simulink model "sfun_daq"  (Simulink 8.3)
settings: Solver=FixedStepDiscrete  StartTime=0.0  StopTime=inf  FixedStep=1/100  RelTol=1e-3
libraries: aerolibtransform2 x1, robotica_R2013b x1
settings Model: Creator=blazj  LastModifiedBy=blazj
settings DataIOCC: SignalLoggingSaveFormat=Dataset
settings DebuggingCC: UnderspecifiedInitializationDetection=Simplified  StateNameClashWarn=none
settings GRTTargetCC: CombineOutputUpdateFcns=on  GRTInterface=off

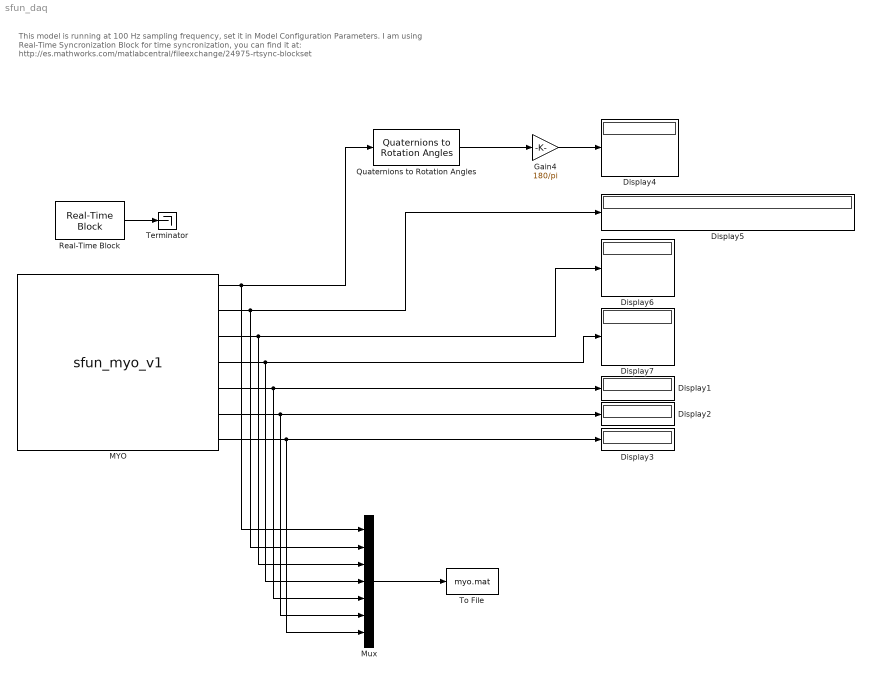
== system sfun_daq ==
  note: This model is running at 100 Hz sampling frequency, set it in Model Configuration Parameters.
      | I am using Real-Time Syncronization Block for time syncronization, you can find it at: http://es.mathworks.com/matlabcentral/fileexchange/24975-rtsync-blockset
  Display{1..7} (7 alike) : Display
  Gain4 : Gain  Gain=180/pi
  MYO : S-Function  FunctionName=sfun_myo_v1  Parameters=1  EnableBusSupport=off
      mask Display:
      | image('myo.jpg')
      | 
      | port_label('output', 1, 'q')
      | port_label('output', 2, 'emg')
      | port_label('output', 3, 'gyro')
      | port_label('output', 4, 'acc')
      | port_label('output', 5, 'pose')
      | port_label('output', 6, 'sync')
      | port_label('output', 7, 'arm')
  Mux : Mux  Inputs=7
  Quaternions to Rotation Angles : aerolibtransform2/Quaternions to Rotation Angles  rotationOrder=ZYX
  Real-Time Block : robotica_R2013b/Utilities blocks/Real-Time Block  sync_type=Fixed  sync_time=1/100
  Terminator : Terminator
  To File : ToFile  Filename=myo.mat  MatrixName=myo  SaveFormat=Timeseries
  wires:
  Quaternions to Rotation Angles/1 -> Gain4/1
  Gain4/1 -> Display4/1
  MYO/1 -> Mux/1, Quaternions to Rotation Angles/1
  MYO/2 -> Mux/2, Display5/1
  MYO/3 -> Mux/3, Display6/1
  MYO/4 -> Mux/4, Display7/1
  MYO/5 -> Mux/5, Display1/1
  MYO/6 -> Mux/6, Display2/1
  MYO/7 -> Mux/7, Display3/1
  Real-Time Block/1 -> Terminator/1
  Mux/1 -> To File/1
